simulink model "straight_level"  (R2016a)
settings: Solver=VariableStepAuto  StartTime=0.0  StopTime=100  RelTol=1e-3
undefined symbols (not defined in the file or in its folder): U_trim, X_trim
libraries: X8_lib x1
settings Model: Creator=andreanv  LastModifiedBy=andreanv

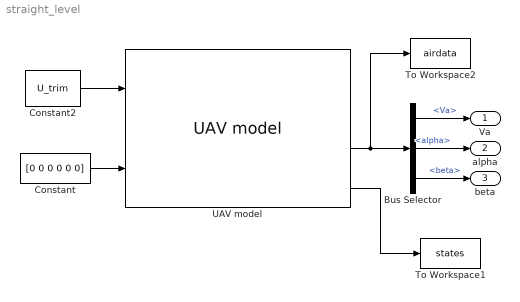
== system straight_level ==
  Bus Selector : BusSelector  OutputSignals=Va,alpha,beta
  Constant : Constant  Value=[0 0 0 0 0 0]
  Constant2 : Constant  Value=U_trim
  To Workspace1 : ToWorkspace  VariableName=states  SaveFormat=Timeseries  SampleTime=-1
  To Workspace2 : ToWorkspace  VariableName=airdata  SaveFormat=Timeseries  SampleTime=-1
  UAV model : X8_lib/UAV model  param=param  pos0=X_trim(1:3)'  quat0=X_trim(4:7)'  vel0=X_trim(8:10)'  rate0=X_trim(11:13)'  servoR_pos0=X_trim(14)  servoR_vel0=X_trim(15)  servoL_pos0=X_trim(16)  servoL_vel0=X_trim(17)  motor_speed0=X_trim(18)
  Va : Outport
  alpha : Outport  Port=2
  beta : Outport  Port=3
  wires:
  Constant/1 -> UAV model/2
  UAV model/3 -> To Workspace2/1, Bus Selector/1
  Bus Selector/1 -> Va/1  "<Va>"
  Bus Selector/2 -> alpha/1  "<alpha>"
  Bus Selector/3 -> beta/1  "<beta>"
  UAV model/4 -> To Workspace1/1
  Constant2/1 -> UAV model/1
